simulink model "magnetorquer_assembly_lib_2"  (R2016b)
settings: Solver=VariableStepAuto  StartTime=0.0  StopTime=10.0  RelTol=1e-3
undefined symbols (not defined in the file): sim_params
libraries: simulink x3
settings Model: Creator=taylorreynolds  LastModifiedBy=taylorreynolds

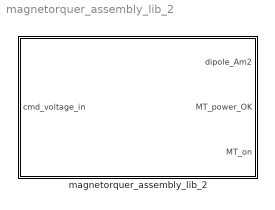
== system magnetorquer_assembly_lib_2 ==
  magnetorquer_assembly_lib_2 : Subsystem

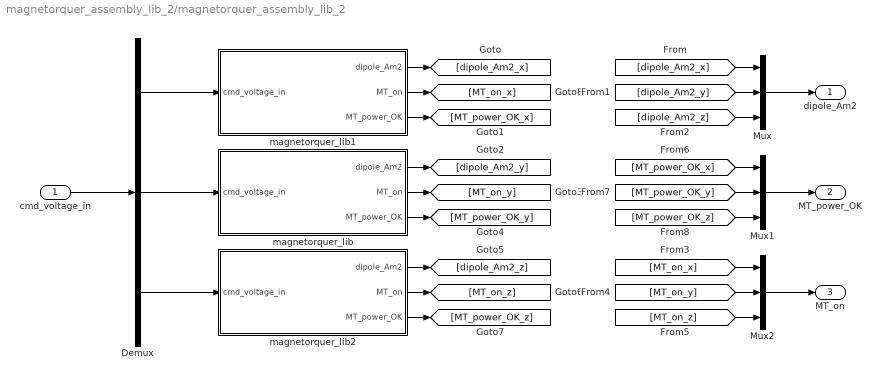
== system magnetorquer_assembly_lib_2/magnetorquer_assembly_lib_2 ==
  cmd_voltage_in : Inport
  Demux : Demux  Outputs=3
  Mux : Mux  Inputs=3
  Mux1 : Mux  Inputs=3
  Mux2 : Mux  Inputs=3
  magnetorquer_lib : Subsystem  mask{voltage_to_dipole=0.25*sim_params.actuators.magnetorquer.max_dipole_y, upperbound=sim_params.actuators.magnetorquer.max_dipole_y, lowerbound=-sim_params.actuators.magnetorquer.max_dipole_y}
      mask prompts: voltage_to_dipole "Simulink:blkprm_prompts:GainGain"; upperbound "Simulink:masks:UpperBound_MP"; lowerbound "Simulink:masks:LowerBound_MP"
      mask TypeOptions voltage_to_dipole: Gain/Gain
      mask TypeOptions upperbound:
      | Check
      | Static Range/max
      mask TypeOptions lowerbound:
      | Check
      | Static Range/min
  magnetorquer_lib1 : Subsystem  mask{voltage_to_dipole=0.25*sim_params.actuators.magnetorquer.max_dipole_x, upperbound=sim_params.actuators.magnetorquer.max_dipole_x, lowerbound=-sim_params.actuators.magnetorquer.max_dipole_x}
      mask prompts: voltage_to_dipole "Simulink:blkprm_prompts:GainGain"; upperbound "Simulink:masks:UpperBound_MP"; lowerbound "Simulink:masks:LowerBound_MP"
      mask TypeOptions voltage_to_dipole: Gain/Gain
      mask TypeOptions upperbound:
      | Check
      | Static Range/max
      mask TypeOptions lowerbound:
      | Check
      | Static Range/min
  magnetorquer_lib2 : Subsystem  mask{voltage_to_dipole=0.25*sim_params.actuators.magnetorquer.max_dipole_z, upperbound=sim_params.actuators.magnetorquer.max_dipole_z, lowerbound=-sim_params.actuators.magnetorquer.max_dipole_z}
      mask prompts: voltage_to_dipole "Simulink:blkprm_prompts:GainGain"; upperbound "Simulink:masks:UpperBound_MP"; lowerbound "Simulink:masks:LowerBound_MP"
      mask TypeOptions voltage_to_dipole: Gain/Gain
      mask TypeOptions upperbound:
      | Check
      | Static Range/max
      mask TypeOptions lowerbound:
      | Check
      | Static Range/min
  dipole_Am2 : Outport
  MT_power_OK : Outport  Port=2
  MT_on : Outport  Port=3
  wires:
  cmd_voltage_in/1 -> Demux/1
  Demux/3 -> magnetorquer_lib2/1(cmd_voltage_in)
  Demux/1 -> magnetorquer_lib1/1(cmd_voltage_in)
  Demux/2 -> magnetorquer_lib/1(cmd_voltage_in)
  magnetorquer_lib1/1(dipole_Am2) -> [dipole_Am2_x]
  magnetorquer_lib2/3(MT_power_OK) -> [MT_power_OK_z]
  magnetorquer_lib2/2(MT_on) -> [MT_on_z]
  magnetorquer_lib2/1(dipole_Am2) -> [dipole_Am2_z]
  magnetorquer_lib/3(MT_power_OK) -> [MT_power_OK_y]
  magnetorquer_lib/2(MT_on) -> [MT_on_y]
  magnetorquer_lib/1(dipole_Am2) -> [dipole_Am2_y]
  magnetorquer_lib1/3(MT_power_OK) -> [MT_power_OK_x]
  magnetorquer_lib1/2(MT_on) -> [MT_on_x]
  Mux/1 -> dipole_Am2/1
  Mux1/1 -> MT_power_OK/1
  Mux2/1 -> MT_on/1
  [dipole_Am2_x] -> Mux/1
  [dipole_Am2_y] -> Mux/2
  [dipole_Am2_z] -> Mux/3
  [MT_on_x] -> Mux2/1
  [MT_on_y] -> Mux2/2
  [MT_on_z] -> Mux2/3
  [MT_power_OK_x] -> Mux1/1
  [MT_power_OK_y] -> Mux1/2
  [MT_power_OK_z] -> Mux1/3

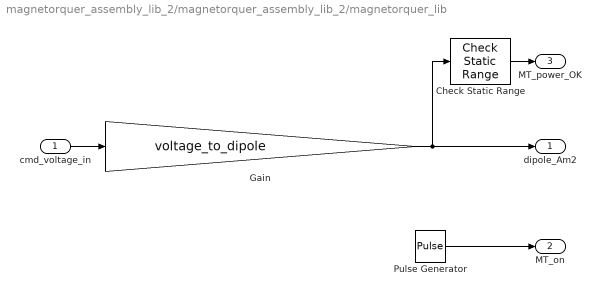
== system magnetorquer_assembly_lib_2/magnetorquer_assembly_lib_2/magnetorquer_lib ==
  cmd_voltage_in : Inport
  Check Static Range : simulink/Model Verification/Check  Static Range  Description=lowerbound <= u <= upperbound  max=upperbound  max_included=on  min=lowerbound  min_included=on  enabled=on  stopWhenAssertionFail=off  export=on  icon=graphic
  Gain : Gain  Gain=voltage_to_dipole
  Pulse Generator : DiscretePulseGenerator  PulseType=Time based  Period=1  PulseWidth=fsw_params.actuators.magnetorquer.actuation_time_pct
  dipole_Am2 : Outport
  MT_on : Outport  Port=2
  MT_power_OK : Outport  Port=3
  wires:
  cmd_voltage_in/1 -> Gain/1
  Gain/1 -> Check Static Range/1, dipole_Am2/1
  Pulse Generator/1 -> MT_on/1
  Check Static Range/1 -> MT_power_OK/1

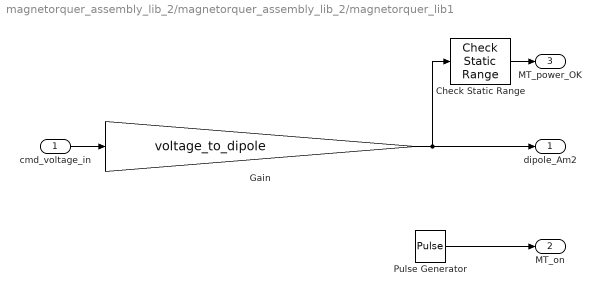
== system magnetorquer_assembly_lib_2/magnetorquer_assembly_lib_2/magnetorquer_lib1 ==
  cmd_voltage_in : Inport
  Check Static Range : simulink/Model Verification/Check  Static Range  Description=lowerbound <= u <= upperbound  max=upperbound  max_included=on  min=lowerbound  min_included=on  enabled=on  stopWhenAssertionFail=off  export=on  icon=graphic
  Gain : Gain  Gain=voltage_to_dipole
  Pulse Generator : DiscretePulseGenerator  PulseType=Time based  Period=1  PulseWidth=fsw_params.actuators.magnetorquer.actuation_time_pct
  dipole_Am2 : Outport
  MT_on : Outport  Port=2
  MT_power_OK : Outport  Port=3
  wires:
  cmd_voltage_in/1 -> Gain/1
  Gain/1 -> Check Static Range/1, dipole_Am2/1
  Pulse Generator/1 -> MT_on/1
  Check Static Range/1 -> MT_power_OK/1

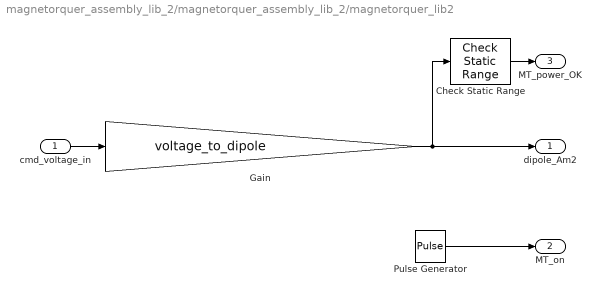
== system magnetorquer_assembly_lib_2/magnetorquer_assembly_lib_2/magnetorquer_lib2 ==
  cmd_voltage_in : Inport
  Check Static Range : simulink/Model Verification/Check  Static Range  Description=lowerbound <= u <= upperbound  max=upperbound  max_included=on  min=lowerbound  min_included=on  enabled=on  stopWhenAssertionFail=off  export=on  icon=graphic
  Gain : Gain  Gain=voltage_to_dipole
  Pulse Generator : DiscretePulseGenerator  PulseType=Time based  Period=1  PulseWidth=fsw_params.actuators.magnetorquer.actuation_time_pct
  dipole_Am2 : Outport
  MT_on : Outport  Port=2
  MT_power_OK : Outport  Port=3
  wires:
  cmd_voltage_in/1 -> Gain/1
  Gain/1 -> Check Static Range/1, dipole_Am2/1
  Pulse Generator/1 -> MT_on/1
  Check Static Range/1 -> MT_power_OK/1
